simulink model "btp8thsemmodel"  (R2024b)
settings: Solver=ode23t  StartTime=0.0  StopTime=10  RelTol=1e-3
libraries: spsControlledVoltageSourceLib x1, spsCurrentMeasurementLib x1, spsGroundLib x1, spsPVArrayLib x1, simulink x1, spsVoltageMeasurementLib x1, sps_lib x1
settings Model: Creator=amsh9  LastModifiedBy=amsh9

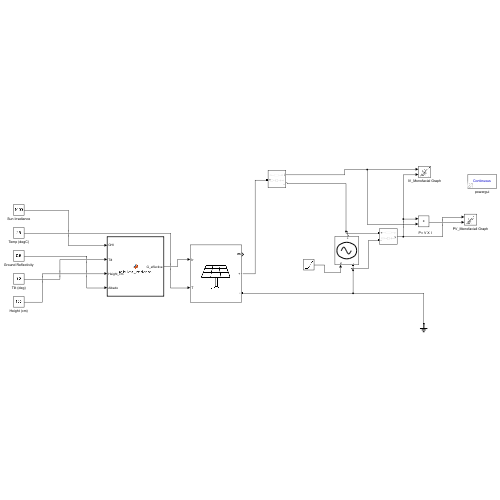
[thumbnail: Simulink's stored preview of the top-level diagram]
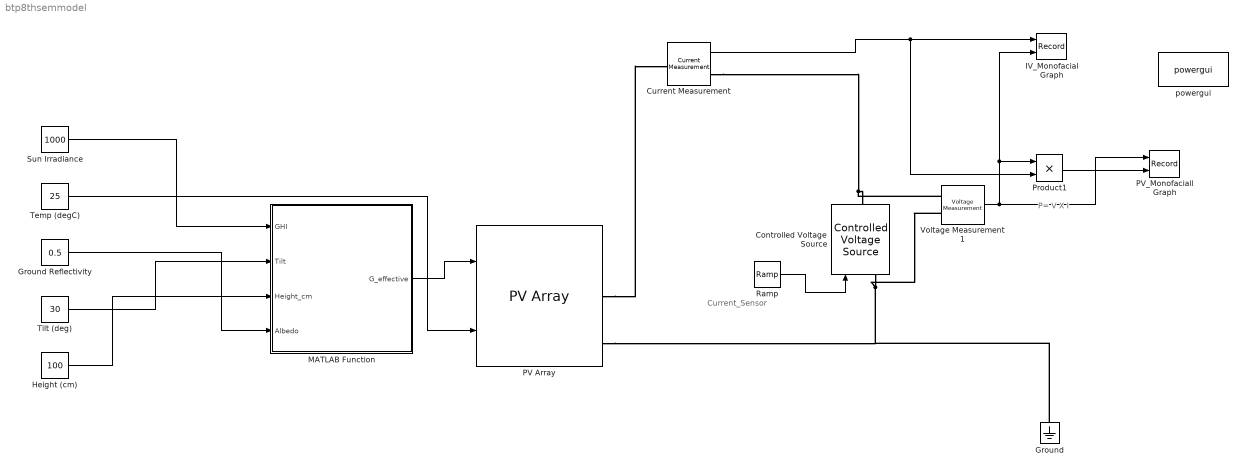
== system btp8thsemmodel ==
  note: P= V X I
  note: Current_Sensor
  Controlled Voltage Source : spsControlledVoltageSourceLib/Controlled Voltage Source  Initialize=on  Source_Type=DC  Amplitude=0  Phase=0  Frequency=0  Measurements=None
  Current Measurement : spsCurrentMeasurementLib/Current Measurement  PhasorSimulation=off  OutputType=Complex  PSBequivalent=0
  Ground : spsGroundLib/Ground  LConnTagsString=a
  Ground Reflectivity : Constant  Value=0.5
  Height (cm) : Constant  Value=100
  IV_Monofacial Graph : Record  FileSettingsInternal="{\"entries\":[{\"content\":{\"excelSettings\":{\"content\":{},\"type\":\"Streamout.ExcelSettings\"}},\"type\":\"Streamout.FileSettingStorage\",\"uuid\":\"\"}],\"packageUris\":[\"http:\\/\\/schema.mathworks.com\\/mf0\\/streamout_blocks\\/R2020a\"],\"version\":\"1.0\"}"  Layout=[1 1]  SignalsInternal="{\"entries\":[{\"content\":{\"signals\":[{\"content\":{\"blockPath\":[],\"dimensions\":[1],\"domain\":\"\",\"lineColor\":\"#a2142f\",\"lineWidth\":2,\"plots\":[ 1 ],\"port\":1,\"sid\":[\"\"],\"signalID\":1,\"signalName\":\"Current Measurement\"},\"type\":\"RecordBlkView.Signal\",\"uuid\":\"\"},{\"content\":{\"blockPath\":[],\"dimensions\":[1],\"domain\":\"\",\"lineColor\":\"#139fff\",\"lineWidth\":2,\"plots\":[ 1 ],\"port\":2,\"sid\":[\"\"],\"signalID\":2,\"signalName\":\"Voltage Measurement1\"},\"type\":\"RecordBlkView.Signal\",\"uuid\":\"\"}]},\"type\":\"RecordBlkView.InputSignals\",\"uuid\":\"\"}],\"packageUris\":[\"http:\\/\\/schema.mathworks.com\\/mf0\\/streamout_blocks\\/R2020a\"],\"version\":\"1.0\"}"  VisualizationBindings="{\"xyplotplugin\":{\"info\":[{\"series\":[{\"bindingParametersList\":[{\"parameter\":\"X-Axis\",\"signalID\":2,\"signalName\":\"Voltage Measurement1\"},{\"parameter\":\"Y-Axis\",\"signalID\":1,\"signalName\":\"Current Measurement\"},{\"parameter\":\"X-Axis\",\"signalID\":2,\"signalName\":\"Voltage Measurement1\"},{\"parameter\":\"Y-Axis\",\"signalID\":1,\"signalName\":\"Current Measurement\"}],\"seriesID\":0}],\"subplotID\":1}]}}"  CompatibilityTag=XY
  MATLAB Function : MATLAB Function  TreatAsAtomicUnit=on
  PV Array : spsPVArrayLib/PV Array  Npar=1  Nser=1  PlotType=array @ 1000 W/m2 & specified temperatures  S_vec="[ 1000  500  100 ]"  Temp_C_vec="[ 25  ]"  ModuleName=User-defined  PlotWhenSelected=off  Pm=213.15  Ncell=60  Voc=36.3  Isc=7.84  Vm=29  Im=7.35  beta_Voc_pc=-0.36099  alpha_Isc_pc=0.102  beta_Voc=-0.13104  alpha_Isc=0.0079968  IL=7.8654  I0=2.9273e-10  nI=0.98119  Rsh=313.0553  Rs=0.39381  RobustModel=off  RobustCellTemperature=313.3991  BAL=on  Tc=1e-6  Tfilter=5e-5
  PV_Monofaciall Graph : Record  FileSettingsInternal="{\"entries\":[{\"content\":{\"excelSettings\":{\"content\":{},\"type\":\"Streamout.ExcelSettings\"}},\"type\":\"Streamout.FileSettingStorage\",\"uuid\":\"\"}],\"packageUris\":[\"http:\\/\\/schema.mathworks.com\\/mf0\\/streamout_blocks\\/R2020a\"],\"version\":\"1.0\"}"  Layout=[1 1]  SignalsInternal="{\"entries\":[{\"content\":{\"signals\":[{\"content\":{\"blockPath\":[],\"dimensions\":[1],\"domain\":\"\",\"lineColor\":\"#a2142f\",\"lineWidth\":2,\"plots\":[ 1 ],\"port\":1,\"sid\":[\"\"],\"signalID\":1,\"signalName\":\"Voltage Measurement1\"},\"type\":\"RecordBlkView.Signal\",\"uuid\":\"\"},{\"content\":{\"blockPath\":[],\"dimensions\":[1],\"domain\":\"\",\"lineColor\":\"#139fff\",\"plots\":[ 1 ],\"port\":2,\"sid\":[\"\"],\"signalID\":2,\"signalName\":\"Product1\"},\"type\":\"RecordBlkView.Signal\",\"uuid\":\"\"}]},\"type\":\"RecordBlkView.InputSignals\",\"uuid\":\"\"}],\"packageUris\":[\"http:\\/\\/schema.mathworks.com\\/mf0\\/streamout_blocks\\/R2020a\"],\"version\":\"1.0\"}"  VisualizationBindings="{\"xyplotplugin\":{\"info\":[{\"series\":[{\"bindingParametersList\":[{\"parameter\":\"X-Axis\",\"signalID\":1,\"signalName\":\"Voltage Measurement1\"},{\"parameter\":\"Y-Axis\",\"signalID\":2,\"signalName\":\"Product1\"},{\"parameter\":\"X-Axis\",\"signalID\":1,\"signalName\":\"Voltage Measurement1\"},{\"parameter\":\"Y-Axis\",\"signalID\":2,\"signalName\":\"Product1\"}],\"seriesID\":0}],\"subplotID\":1}]}}"  CompatibilityTag=XY
  Product1 : Product
  Ramp : simulink/Sources/Ramp  slope=10  start=0  InitialOutput=0
  Sun Irradiance : Constant  Value=1000
  Temp (degC) : Constant  Value=25
  Tilt (deg) : Constant  Value=30
  Voltage Measurement1 : spsVoltageMeasurementLib/Voltage Measurement  PhasorSimulation=off  OutputType=Complex  PSBequivalent=0
  powergui : sps_lib/powergui  Priority=1  SimulationMode=Continuous  SampleTime=50e-6  frequency=60  Iterations=50  frequencyindice=0  Pbase=100e6  ErrMax=1e-4  UnitsV=kV  UnitsW=MW  buscounter=0  FunctionMessages=off  echomessages=off  EnableUseOfTLC=off  CurrentSourceSwitches=off  DisableSnubberDevices=off  DisableRonSwitches=off  DisableVfSwitches=off  DisplayEquations=off  AutomaticDiscreteSolvers=off  SolverType=Tustin/Backward Euler (TBE)  Interpol=off  ExternalGateDelay=off  methode=off  Ts=100  x0status=blocks  SPID=on  SwTol=0  HookPort=off  NonlinearTolerance=1e-4  nMaxIteration=100  ContinueOnMaxIteration=off  RestoreLinks=warning  ResistiveCurrentMeasurement=off  Frange=[0:2:500]  Ylog=off  Xlog=on  ShowGrid=off  save=off  variable=ZData  structure=0  ZoomFFT=off  StartTime=0.0  cycles=1  DisplayStyle=1  fundamental=60  FreqAxis=off  MaxFrequency=1000  frequencyindicesteady=1  RmsSteady=1  display=off
  wires:
  Product1/1 -> PV_Monofaciall Graph/2
  Height (cm)/1 -> MATLAB Function/3(Height_cm)
  Tilt (deg)/1 -> MATLAB Function/2(Tilt)
  Ground Reflectivity/1 -> MATLAB Function/4(Albedo)
  Sun Irradiance/1 -> MATLAB Function/1(GHI)
  MATLAB Function/1(G_effective) -> PV Array/1
  Temp (degC)/1 -> PV Array/2
  Ramp/1 -> Controlled Voltage Source/1
  Voltage Measurement1/1 -> PV_Monofaciall Graph/1, Product1/1, IV_Monofacial Graph/2
  Current Measurement/1 -> Product1/2, IV_Monofacial Graph/1
  connections:
  PV Array/RConn1 -- Current Measurement/LConn1
  Current Measurement/RConn1 -- Voltage Measurement1/LConn1 -- Controlled Voltage Source/RConn1
  Controlled Voltage Source/LConn1 -- Ground/LConn1 -- PV Array/RConn2 -- Voltage Measurement1/LConn2

== matlab function btp8thsemmodel/MATLAB Function ==
  data: GHI input; Tilt input; Height_cm input; G_effective output; Albedo input
function G_effective = calculate_irradiance(GHI, Tilt, Height_cm,Albedo)
    % 1. View Factor (Geometric logic)
    beta_rad = deg2rad(Tilt);
    View_Factor = (1 - cos(beta_rad)) / 2;
    
    % 2. Height Factor (Dincer et al. 2025)
    H_Factor = (1 + (Height_cm / 1000));
    
    % 3. Calculate Rear Irradiance (W/m2)
    G_rear_raw = GHI * Albedo * View_Factor * H_Factor;
    
    % 4. Apply Bifaciality Factor (70% efficiency on rear)
    Bifaciality = 0.7; 
    G_rear_effective = G_rear_raw * Bifaciality;
    
    % 5. Total Effective Irradiance (Input for PV Array)
    % This sums the front sun + the rear contribution
    G_effective = GHI + G_rear_effective;
end
